simulink model "Mixed_Radix_FFT_Ex2"  (R2022a)
settings: Solver=VariableStepAuto  StartTime=0.0  StopTime=1  RelTol=1e-3
undefined symbols (not defined in the file): None, Radix, S, vsva2197, xcvc1902
libraries: dspsrcs4 x1, aieDSP x1, dspxfrm3 x1, vmcUtilities x1
settings Model: Creator=sdegala  LastModifiedBy=sdegala

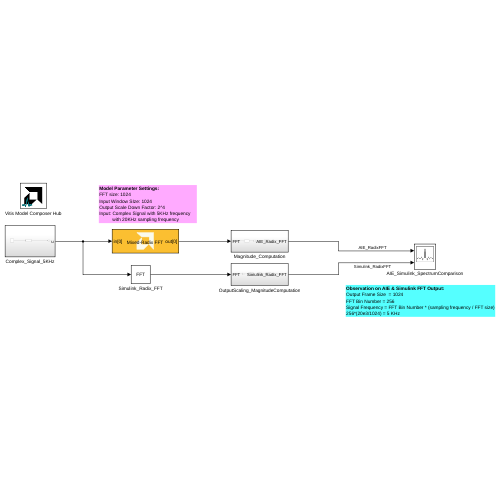
[thumbnail: Simulink's stored preview of the top-level diagram]
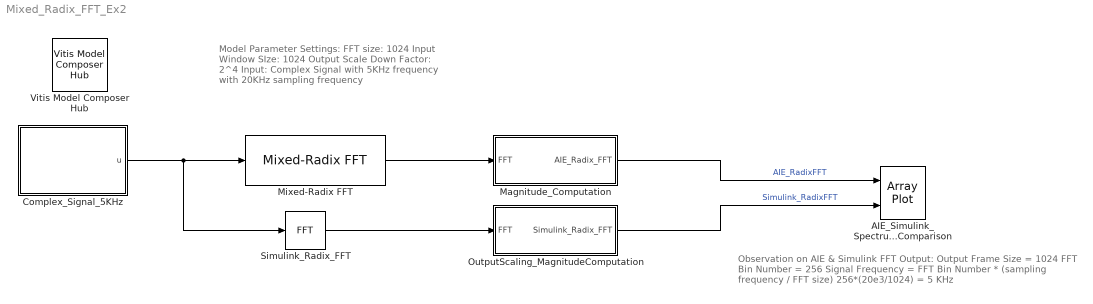
== system Mixed_Radix_FFT_Ex2 ==
  note: Observation on AIE & Simulink FFT Output:
      | Output Frame Size = 1024
      | FFT Bin Number = 256
      | Signal Frequency = FFT Bin Number * (sampling frequency / FFT size)
      | 256*(20e3/1024) = 5 KHz
  note: Model Parameter Settings:
      | FFT size: 1024
      | Input Window SIze: 1024
      | Output Scale Down Factor: 2^4
      | Input: Complex Signal with 5KHz frequency
      | with 20KHz sampling frequency
  AIE_Simulink_SpectrumComparison : ArrayPlot  NumInputPorts=2  WindowPosition=[83.000000,69.000000,1116.000000,539.000000,]  ScopeFrameLocation=window  PlotType=Line  AxesScaling=Manual  YLimits=[-10,100]  ShowLegend=on
  Complex_Signal_5KHz : Subsystem
  Magnitude_Computation : Subsystem
  Mixed-Radix FFT : aieDSP/Mixed-Radix FFT  data_type=cint16  twiddle_type=cint16  point_size=1024  input_window_size=1024  shift_val=4  rnd_mode=Round symmetrical to infinity  sat_mode=0-None  casc_length=1  blockJsonConstraints=[]  blockJsonConstraintsInternal=[]  spec=vmc_mixed_radix_fft.json  SerializedMaskParamNames=[]  SerializedMaskParamValues=[]  SerializedMaskParamVisibilities=[]  block_type=Mixed-Radix FFT  SerializedMaskParamDataypes=typename|typename|uint|uint|uint|uint|uint|uint  SerializedMaskParamEnumStrArr=0|0|0|0|0|Floor,Ceiling,Round to positive infinity,Round to negative infinity,Round symmetrical to infinity,Round symmetrical to zero,Round convergent to even,Round convergent to odd|0-None,1-Asymmetric,3-Symmetric|0  SerializedMaskParamEnumValArr=0|0|0|0|0|0,1,2,3,4,5,6,7|0,1,3|0  SerializedMaskParamVectorArr=0|0|0|0|0|0|0|0
  OutputScaling_MagnitudeComputation : Subsystem
  Simulink_Radix_FFT : dspxfrm3/FFT  FFTImplementation=Radix-2  CompMethod=Table lookup  TableOpt=NEW  TableOptActive=Speed  BitRevOrder=off  Normalize=off  InheritFFTLength=on  FFTLength=8  WrapInput=on  roundingMode=Floor  overflowMode=off  firstCoeffDataTypeStr=Inherit: Same word length as input  firstCoeffLastDataTypeStr=Inherit: Same word length as input  prodOutputMode=Binary point scaling  prodOutputWordLength=24  prodOutputFracLength=0  prodOutputDataTypeStr=fixdt(1,24,0)  prodOutputLastDataTypeStr=fixdt(1,24,0)  accumMode=Binary point scaling  accumWordLength=28  accumFracLength=0  accumDataTypeStr=fixdt(1,28,0)  accumLastDataTypeStr=fixdt(1,28,0)  outputMode=Binary point scaling  outputWordLength=16  outputFracLength=0  outputDataTypeStr=fixdt(1,16,0)  outputMin=[]  outputMax=[]  outputLastDataTypeStr=fixdt(1,16,0)
  Vitis Model Composer Hub : vmcUtilities/Vitis Model Composer Hub  Tag=genX  CodeGeneration=off  TargetDirectory=./code  ExportType=AI Engines  IpVendor=xilinx.com  IpLibrary=hls  IpVersion=1.0  IpHWLanguage=Verilog  AieCompilerOptions={}  AieSimulatorOptions={}  CreateTestbench=off  TestbenchStackSize=10  RunRtlSim=off  RunCSim=off  RunAieSim=off  AieSimTimeout=50000  RunAieSimProfiling=off  LaunchVitisAnalyzer=off  PlotOutput=off  RunX86Sim=off  X86SimTimeout=10  GenHwImage=off  GenLibadfXo=off  PlatformType=Not Specified  HwSystemType=Baremetal  HwValidationTarget=hw  ProjDevice=xcvc1902-vsva2197-1LP-e-S  ProjDevicePart=xcvc1902-vsva2197-1LP-e-S  AIEType=AIE  SamplePeriod=-1  ClockFrequency=200  DataPathParallelism=1  xilinxfamily=versalaicore  part=xcvc1902  speed=-1LP-e-S  package=vsva2197  directory=./netlist  testbench=off  incr_netlist=off  synthesis_tool=Vivado  clock_wrapper=Clock Enables  dbl_ovrd=According to Block Masks  dcm_input_clock_period=10  sysclk_period=10  simulink_period=1  eval_field=0  LogFileName=''  NThreads=4
  wires:
  Simulink_Radix_FFT/1 -> OutputScaling_MagnitudeComputation/1(FFT)
  Mixed-Radix FFT/1 -> Magnitude_Computation/1(FFT)
  Complex_Signal_5KHz/1(u) -> Mixed-Radix FFT/1, Simulink_Radix_FFT/1
  Magnitude_Computation/1(AIE_Radix_FFT) -> AIE_Simulink_SpectrumComparison/1  "AIE_RadixFFT"
  OutputScaling_MagnitudeComputation/1(Simulink_Radix_FFT) -> AIE_Simulink_SpectrumComparison/2  "Simulink_RadixFFT"

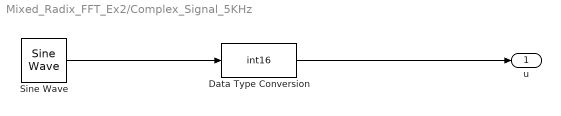
== system Mixed_Radix_FFT_Ex2/Complex_Signal_5KHz ==
  Data Type Conversion : DataTypeConversion  OutDataTypeStr=int16  SaturateOnIntegerOverflow=off  RndMeth=Floor
  Sine Wave : dspsrcs4/Sine Wave  Amplitude=1  Frequency=5e3  Phase=0  SampleMode=Discrete  OutComplex=Complex  CompMethod=Table lookup  TableSize=Speed  SampleTime=1/20e3  SamplesPerFrame=1024  ResetState=Restart at time zero  OutputFrames=off  dataType=Fixed-point  wordLen=16  udDataType=sfix(16)  fracBitsMode=User-defined  numFracBits=14  OutDataTypeStr=fixdt(1,16,14)  LastOutDataTypeStr=fixdt(1,16,14)
  u : Outport
  wires:
  Sine Wave/1 -> Data Type Conversion/1
  Data Type Conversion/1 -> u/1

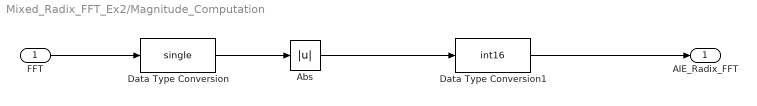
== system Mixed_Radix_FFT_Ex2/Magnitude_Computation ==
  FFT : Inport
  Abs : Abs  SaturateOnIntegerOverflow=off
  Data Type Conversion : DataTypeConversion  OutDataTypeStr=single  SaturateOnIntegerOverflow=off  RndMeth=Floor
  Data Type Conversion1 : DataTypeConversion  OutDataTypeStr=int16  SaturateOnIntegerOverflow=off  RndMeth=Floor
  AIE_Radix_FFT : Outport
  wires:
  Data Type Conversion/1 -> Abs/1
  FFT/1 -> Data Type Conversion/1
  Abs/1 -> Data Type Conversion1/1
  Data Type Conversion1/1 -> AIE_Radix_FFT/1

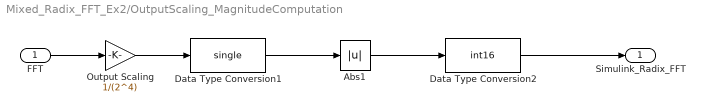
== system Mixed_Radix_FFT_Ex2/OutputScaling_MagnitudeComputation ==
  FFT : Inport
  Abs1 : Abs  SaturateOnIntegerOverflow=off
  Data Type Conversion1 : DataTypeConversion  OutDataTypeStr=single  SaturateOnIntegerOverflow=off  RndMeth=Floor
  Data Type Conversion2 : DataTypeConversion  OutDataTypeStr=int16  SaturateOnIntegerOverflow=off  RndMeth=Floor
  "Output Scaling " : Gain  Gain=1/(2^4)
  Simulink_Radix_FFT : Outport
  wires:
  Data Type Conversion1/1 -> Abs1/1
  Abs1/1 -> Data Type Conversion2/1
  FFT/1 -> "Output Scaling "/1
  Data Type Conversion2/1 -> Simulink_Radix_FFT/1
  "Output Scaling "/1 -> Data Type Conversion1/1
